simulink model "ExoskeletonControlModel"  (R2022b)
settings: Solver=ode3  StartTime=0.0  StopTime=inf  FixedStep=Ts  RelTol=1e-3
PreLoadFcn:
  | Ts_IO204 = 0.001;
  | 
  | if ~exist('Ts', 'var')
  | Ts = 0.001;
  | end
  | if ~exist('FPGA_Frequency', 'var')
  | FPGA_Frequency = 75000000;
  | end
  | 
  | ts_IO612 = 1e-3;
  | 
  | load('TargetReached.mat')
  | load('ActualPos_inc.mat')
model workspace (MAT data in the model file):
  DeltaData : timeseries (value not decoded)
  EC45_deg2incs = 2276
  EC60_deg2inc = 5461
  EC90_deg2incs = 7111
  Enc2rad_18bit = 2.3968e-05
  Enc2rad_19bit = 1.1984e-05
  Enc2rad_20bit = 5.9921e-06
  GiulioModel : robotics.RigidBodyTree (value not decoded)
  Giulio_Spheric_model : robotics.RigidBodyTree (value not decoded)
  Offset1_ticks = 571315
  Offset2_ticks = 590938.9928
  Offset3_ticks = 457912.8279
  Offset4_ticks = 482293.9763
  Offset5_ticks = 598735.9316
  Offset_M1 = 1.12645499896
  Offset_M2 = 4.02728553608
  Offset_M3 = 5.48587511336
  Offset_M4 = 2.03717511516
  Offset_M5 = 4.4996674016
  T1_Nm : object (value not decoded)
  T2_Nm : object (value not decoded)
  TBmodel : robotics.RigidBodyTree (value not decoded)
  Ts = 0.002
  Xg : object (value not decoded)
  Yg : object (value not decoded)
  Zg : object (value not decoded)
  a2 = 0.27
  change_variable = 0
  d1 = [0 0 0 0 0 0 0 0 0 0 0 0 ... (30001 elements, 30001x1)]
  d1_1 = 0.21074
  d2 = [0 0 0 0 0 0 0 0 0 0 0 0 ... (30001 elements, 30001x1)]
  d2_1 = 0.04864
  d3 = [0 0 0 0 0 0 0 0 0 0 0 0 ... (30001 elements, 30001x1)]
  d4 = [0 0 0 0 0 0 0 0 0 0 0 0 ... (30001 elements, 30001x1)]
  d5 = [0 0 0 0 0 0 0 0 0 0 0 0 ... (30001 elements, 30001x1)]
  d6 = [0 0 0 0 0 0 0 0 0 0 0 0 ... (30001 elements, 30001x1)]
  ee_x = -0.2852
  ee_y = -0.3683
  ee_z = -0.0386
  enc2rad_EC45 = 7.6699e-06
  enc2rad_EC90 = 2.3969e-05
  k1_Nm_ticks = 0.00923
  k2_Nm_ticks = 0.0257
  k3_Nm_ticks = 0.00692
  k4_Nm_ticks = 0.00729
  k5_Nm_ticks = 0.00641
  lower_lim_m1 = -330000
  lower_lim_m2 = -235302
  lower_lim_m3 = -132865
  lower_lim_m4 = -152732
  lower_lim_m5 = -138363
  lower_lim_m6 = -200325
  m1 = 2.441408578
  m2 = 3.750007
  m3 = 1.56250298
  m4 = 1.56250298
  m5 = 1.56250298
  m6 = 1.56250298
  n_oversampling = 8
  offset_sea_1 = 0.5547
  offset_sea_2 = 2.8595
  offset_sea_3 = 3.5058
  offset_sea_4 = 2.8586
  offset_sea_5 = 2.8736
  params : AKSIM (value not decoded)
  pos_th_neg = -180000
  pos_th_pos = 180000
  q1 = -1819347
  q2 = -196752
  q3 = -596465
  q4 = -556807
  q5 = -573932
  q6 = -489063
  sine = [0 0.187999937334 0.751998997352 1.69199492401 3.0079839574 4.6999608335 6.76791878442 9.21184953835 12.0317433196 15.2275888485 18.7993733417 22.7470825122 ... (12501 elements, 12501x1)]
  start : object (value not decoded)
  switch_admittance = 1
  t1 : object (value not decoded)
  t2 : object (value not decoded)
  torsionalStiffnes_M1 = 384.88
  torsionalStiffnes_M2 = 1500
  torsionalStiffnes_M3 = 901.97
  torsionalStiffnes_M4 = 950.86
  torsionalStiffnes_M5 = 930
  torsionalStiffnes_M6 = 914
  upper_lim_m1 = 340000
  upper_lim_m2 = 95467
  upper_lim_m3 = 164951
  upper_lim_m4 = 210607
  upper_lim_m5 = 252595
  upper_lim_m6 = 96694
  vel_th_neg = -100
  vel_th_pos = 100
  x = 0
undefined symbols (not defined in the file): C, DiscIntNeverNeededParam
libraries: canmsglib x285, speedgoatlib_IO614 x245, simulink x26, slrealtimeloglib x9, simulink_extras x6, robotmaniplib x6
(part 12 of 13)

== stateflow chart ExoskeletonControlModel/DataProcessing/Working_Chart ==
  state Sleep
    en:
    Working_Chart_state=1
    EnableCST=0
    EnableCSPM5=0
    EnableCSPM6=0
    EnableLR_CSP=0
    goal_m1=0
    goal_m2=0
    goal_m3=0
    goal_m4=0
    goal_m5=0
    goal_m6=0
  state Transparency
    state Block_not_recorded_joints
      state ST1_set_CSP_M1 [parallel]
        settings: executionOrder=1
      state ST1_set_CSP_M6 [parallel]
        settings: executionOrder=2
    state Learn
      state Initialize
        en:
        Working_Chart_state=12
        Spring_m6=0
        Spring_m5=0
        Spring_m4=0
        Spring_m3=0
        i=1;
        buffer5(:,1)=0;
        LearnedMovement5(:,1)=0;
        buffer4(:,1)=0;
        LearnedMovement4(:,1)=0;
        buffer3(:,1)=0;
        LearnedMovement3(:,1)=0;
      state writeRegister
        en:
        LearnedMovement5(k,1)=buffer5(k,1);
        LearnedMovement4(k,1)=buffer4(k,1);
        LearnedMovement3(k,1)=buffer3(k,1);
        mov_lenght=i;
        Working_Chart_state=11
      state Recording
        en:
        Start_m1=1
        Start_m2=1
        Start_m3=1
        Start_m4=1
        Start_m5=1
        Start_m6=1
        Working_Chart_state=4
        buffer5(i,1)=ActualPos_inc.p5;
        buffer4(i,1)=ActualPos_inc.p4;
        buffer3(i,1)=ActualPos_inc.p3;
      (default) -> Initialize
      writeRegister -> writeRegister [order 2] : [after(0.002,sec)]{k=k+1}
      Recording -> writeRegister [order 1] : [(hasChangedTo(Mode_selector,8))||(i>9998)]{k=1}
      Initialize -> Recording : [Mode_selector==7]{EnableCST=1}
      Recording -> Recording [order 2] : [after(0.002,sec)]{i=i+1}
    state TransparencyMode
      state EnablePIDs
        Start_m1=1
        Start_m2=1
        Start_m3=1
        Start_m4=1
        Start_m5=1
        Start_m6=1
      state TransparencyActive
        Working_Chart_state=4
        Spring_m6=0
        Spring_m5=0
        Spring_m4=0
        Spring_m3=0
      state WorkingInTrasparency
      (default) -> TransparencyActive
      Transparency.TransparencyMode.EnablePIDs -> WorkingInTrasparency
      TransparencyActive -> Transparency.TransparencyMode.EnablePIDs : {EnableCST=1}
    state ResetState
    state SET_MODE
      state ST1_set_CST_M1 [parallel]
        settings: executionOrder=1
      state ST1_set_CSP_M2 [parallel]
        settings: executionOrder=2
      state ST1_set_CST_M3 [parallel]
        settings: executionOrder=3
      state ST1_set_CST_M4 [parallel]
        settings: executionOrder=4
      state ST1_set_CST_M5 [parallel]
        settings: executionOrder=5
      state ST1_set_CST_M6 [parallel]
        settings: executionOrder=6
    state ImpedanceMode
      state ShoulderFlexion
        state ST1_set_CSP_M4 [parallel]
          settings: executionOrder=1
        state ST1_set_CSP_M3 [parallel]
          settings: executionOrder=2
        state ST1_set_CSP_M6 [parallel]
          settings: executionOrder=3
      state EnablePIDs
        en:
        reset_count_M5=1
        Start_m1=1
        Start_m2=1
        Start_m3=1
        Start_m4=1
        Start_m5=1
        Start_m6=1
      state WorkingInImpedance
      (default) -> ShoulderFlexion : {Working_Chart_state=5;}
      Transparency.ImpedanceMode.EnablePIDs -> WorkingInImpedance
      ShoulderFlexion -> Transparency.ImpedanceMode.EnablePIDs : {EnableCST=1}
    state L_R_CSP
      en:
      EnableLR_CSP=1;
      Working_Chart_state=13
    state GoToExerciseHome
      Working_Chart_state=6
      EnableCST=0
      EnableCSPM5=0
      EnableCSPM6=0
      EnableLR_CSP=0
      goal_m1=0
      goal_m2=0
      goal_m3=0
      goal_m4=0
      goal_m5=0
      goal_m6=0
      state GoHome_M1 [parallel]
        settings: executionOrder=1
        state ST1_set_PPM_M1
        state ST2_Switch_on_Enable_M1
        state ST3_send_target_pos_M1
        state ST4_Abs_ref_start_immediatly_M1
        state Wait_M1
        state Reached_M1
          goal_m1=1
        (default) -> Transparency.GoToExerciseHome.GoHome_M1.ST1_set_PPM_M1
        Transparency.GoToExerciseHome.GoHome_M1.ST1_set_PPM_M1 -> Transparency.GoToExerciseHome.GoHome_M1.ST2_Switch_on_Enable_M1
        Transparency.GoToExerciseHome.GoHome_M1.ST2_Switch_on_Enable_M1 -> Transparency.GoToExerciseHome.GoHome_M1.ST3_send_target_pos_M1
        Transparency.GoToExerciseHome.GoHome_M1.ST3_send_target_pos_M1 -> Transparency.GoToExerciseHome.GoHome_M1.ST4_Abs_ref_start_immediatly_M1
        Transparency.GoToExerciseHome.GoHome_M1.ST4_Abs_ref_start_immediatly_M1 -> Transparency.GoToExerciseHome.GoHome_M1.Wait_M1
        Transparency.GoToExerciseHome.GoHome_M1.Wait_M1 -> Transparency.GoToExerciseHome.GoHome_M1.Reached_M1 : [TargetReached.m1=="Target reached"]
      state GoHome_M2 [parallel]
        settings: executionOrder=2
        state ST1_set_PPM_M2
        state ST2_Switch_on_Enable_M2
        state ST3_send_target_pos_M2
        state ST4_Abs_ref_start_immediatly_M2
        state Wait_M2
        state Reached_M1
          goal_m2=1
        (default) -> Transparency.GoToExerciseHome.GoHome_M2.ST1_set_PPM_M2
        Transparency.GoToExerciseHome.GoHome_M2.ST1_set_PPM_M2 -> Transparency.GoToExerciseHome.GoHome_M2.ST2_Switch_on_Enable_M2
        Transparency.GoToExerciseHome.GoHome_M2.ST2_Switch_on_Enable_M2 -> Transparency.GoToExerciseHome.GoHome_M2.ST3_send_target_pos_M2
        Transparency.GoToExerciseHome.GoHome_M2.ST3_send_target_pos_M2 -> Transparency.GoToExerciseHome.GoHome_M2.ST4_Abs_ref_start_immediatly_M2
        Transparency.GoToExerciseHome.GoHome_M2.ST4_Abs_ref_start_immediatly_M2 -> Transparency.GoToExerciseHome.GoHome_M2.Wait_M2
        Transparency.GoToExerciseHome.GoHome_M2.Wait_M2 -> Transparency.GoToExerciseHome.GoHome_M2.Reached_M1 : [TargetReached.m2=="Target reached"]
      state GoHome_M3 [parallel]
        settings: executionOrder=3
        state ST1_set_PPM_M3
        state ST2_Switch_on_Enable_M3
        state ST3_send_target_pos_M3
        state ST4_Abs_ref_start_immediatly_M3
        state Wait_M3
        state Reached_M3
          goal_m3=1
        (default) -> Transparency.GoToExerciseHome.GoHome_M3.ST1_set_PPM_M3
        Transparency.GoToExerciseHome.GoHome_M3.ST1_set_PPM_M3 -> Transparency.GoToExerciseHome.GoHome_M3.ST2_Switch_on_Enable_M3
        Transparency.GoToExerciseHome.GoHome_M3.ST2_Switch_on_Enable_M3 -> Transparency.GoToExerciseHome.GoHome_M3.ST3_send_target_pos_M3
        Transparency.GoToExerciseHome.GoHome_M3.ST3_send_target_pos_M3 -> Transparency.GoToExerciseHome.GoHome_M3.ST4_Abs_ref_start_immediatly_M3
        Transparency.GoToExerciseHome.GoHome_M3.ST4_Abs_ref_start_immediatly_M3 -> Transparency.GoToExerciseHome.GoHome_M3.Wait_M3
        Transparency.GoToExerciseHome.GoHome_M3.Wait_M3 -> Transparency.GoToExerciseHome.GoHome_M3.Reached_M3 : [TargetReached.m3=="Target reached"]
      state GoHome_M4 [parallel]
        settings: executionOrder=4
        state ST1_set_PPM_M4
        state ST2_Switch_on_Enable_M4
        state ST3_send_target_pos_M4
        state ST4_Abs_ref_start_immediatly_M4
        state Wait_M4
        state Reached_M4
          goal_m4=1
        state ST3_send_target_pos_M4_abd
        (default) -> Transparency.GoToExerciseHome.GoHome_M4.ST1_set_PPM_M4
        Transparency.GoToExerciseHome.GoHome_M4.ST1_set_PPM_M4 -> Transparency.GoToExerciseHome.GoHome_M4.ST2_Switch_on_Enable_M4
        Transparency.GoToExerciseHome.GoHome_M4.ST2_Switch_on_Enable_M4 -> Transparency.GoToExerciseHome.GoHome_M4.ST3_send_target_pos_M4 [order 1] : [(Mode_selector==4)||(Mode_selector==5)||(Mode_selector==9)]
        Transparency.GoToExerciseHome.GoHome_M4.ST3_send_target_pos_M4 -> (junction 459)
        (junction 459) -> Transparency.GoToExerciseHome.GoHome_M4.ST4_Abs_ref_start_immediatly_M4
        Transparency.GoToExerciseHome.GoHome_M4.ST4_Abs_ref_start_immediatly_M4 -> Transparency.GoToExerciseHome.GoHome_M4.Wait_M4
        Transparency.GoToExerciseHome.GoHome_M4.Wait_M4 -> Transparency.GoToExerciseHome.GoHome_M4.Reached_M4 : [TargetReached.m4=="Target reached"]
        ST3_send_target_pos_M4_abd -> (junction 459)
        Transparency.GoToExerciseHome.GoHome_M4.ST2_Switch_on_Enable_M4 -> ST3_send_target_pos_M4_abd [order 2] : [Mode_selector==6]
      state GoHome_M5 [parallel]
        settings: executionOrder=5
        state ST1_set_PPM_M5
        state ST2_Switch_on_Enable_M5
        state ST3_send_target_pos_M5
        state ST4_Abs_ref_start_immediatly_M5
        state Wait_M5
        state Reached_M5
          goal_m5=1
        (default) -> Transparency.GoToExerciseHome.GoHome_M5.ST1_set_PPM_M5
        Transparency.GoToExerciseHome.GoHome_M5.ST1_set_PPM_M5 -> Transparency.GoToExerciseHome.GoHome_M5.ST2_Switch_on_Enable_M5
        Transparency.GoToExerciseHome.GoHome_M5.ST2_Switch_on_Enable_M5 -> Transparency.GoToExerciseHome.GoHome_M5.ST3_send_target_pos_M5
        Transparency.GoToExerciseHome.GoHome_M5.ST3_send_target_pos_M5 -> Transparency.GoToExerciseHome.GoHome_M5.ST4_Abs_ref_start_immediatly_M5
        Transparency.GoToExerciseHome.GoHome_M5.ST4_Abs_ref_start_immediatly_M5 -> Transparency.GoToExerciseHome.GoHome_M5.Wait_M5
        Transparency.GoToExerciseHome.GoHome_M5.Wait_M5 -> Transparency.GoToExerciseHome.GoHome_M5.Reached_M5 : [TargetReached.m5=="Target reached"]
      state GoHome_M6 [parallel]
        settings: executionOrder=6
        state ST1_set_PPM_M6
        state ST2_Switch_on_Enable_M6
        state ST3_send_target_pos_M6
        state ST4_Abs_ref_start_immediatly_M6
        state Wait_M6
        state Reached_M6
          goal_m6=1
        (default) -> Transparency.GoToExerciseHome.GoHome_M6.ST1_set_PPM_M6
        Transparency.GoToExerciseHome.GoHome_M6.ST1_set_PPM_M6 -> Transparency.GoToExerciseHome.GoHome_M6.ST2_Switch_on_Enable_M6
        Transparency.GoToExerciseHome.GoHome_M6.ST2_Switch_on_Enable_M6 -> Transparency.GoToExerciseHome.GoHome_M6.ST3_send_target_pos_M6
        Transparency.GoToExerciseHome.GoHome_M6.ST3_send_target_pos_M6 -> Transparency.GoToExerciseHome.GoHome_M6.ST4_Abs_ref_start_immediatly_M6
        Transparency.GoToExerciseHome.GoHome_M6.ST4_Abs_ref_start_immediatly_M6 -> Transparency.GoToExerciseHome.GoHome_M6.Wait_M6
        Transparency.GoToExerciseHome.GoHome_M6.Wait_M6 -> Transparency.GoToExerciseHome.GoHome_M6.Reached_M6 : [TargetReached.m6=="Target reached"]
    state LowAssistance
      Spring_m5=13
      Spring_m4=15
      Spring_m3=13
    state Set_CST_M5_ShoulderFlexion1
      Working_Chart_state=13
      state ST1_set_CST_M5 [parallel]
        settings: executionOrder=1
      state ST1_set_CST_M3 [parallel]
        settings: executionOrder=2
      state ST1_set_CST_M4 [parallel]
        settings: executionOrder=3
    state MediumAssistance
      Spring_m5=25
      Spring_m4=20
      Spring_m3=20
    state HighAssistance
      Spring_m5=35
      Spring_m4=30
      Spring_m3=30
    state Set_CST_M5_ShoulderFlexion
      Working_Chart_state=6
      state ST1_set_CST_M5
    state Enable
      en:
      Start_m1=1
      Start_m2=1
      Start_m3=1
      Start_m4=1
      Start_m5=1
      Start_m6=1
    state SetCSPforALL
      state ST1_set_CSP_M1 [parallel]
        settings: executionOrder=1
      state ST1_set_CSP_M2 [parallel]
        settings: executionOrder=2
      state ST1_set_CSP_M3 [parallel]
        settings: executionOrder=3
      state ST1_set_CST_M5 [parallel]
        settings: executionOrder=6
      state ST1_set_CSP_M4 [parallel]
        settings: executionOrder=4
      state ST1_set_CSP_M6 [parallel]
        settings: executionOrder=5
    state LowAssistance2
      Spring_m5=10
    state WIP_Exercise
    state MediumAssistance2
      Spring_m5=30
    state HighAssistance2
      Spring_m5=55
    state ENABLE_RIGID_CONTROL_M5
      en:
      Working_Chart_state=6
      EnableCSPM5=1
      EnableCSPM6=0
    state Set_CST_M6_ElbowFlexion
      Working_Chart_state=7
      state ST1_set_CST_M6
    state ExerciseEnded
    state ENABLE_RIGID_CONTROL_M6
      en:
      Working_Chart_state=7
      EnableCSPM5=0
      EnableCSPM6=1
    state LowAssistance1
      Spring_m6=10
    state MediumAssistance1
      Spring_m6=20
    state HighAssistance1
      Spring_m6=30
    Block_not_recorded_joints -> Learn : {i=1;}
    SET_MODE -> Block_not_recorded_joints [order 1] : [Mode_selector==7]
    (default) -> ResetState
    SET_MODE -> TransparencyMode [order 2] : [Mode_selector==2]
    ResetState -> SET_MODE [order 1] : [(Mode_selector==2)||(Mode_selector==3)||(Mode_selector==7)]
    SET_MODE -> ImpedanceMode [order 3] : [Mode_selector==3]
    ResetState -> GoToExerciseHome [order 2] : [(Mode_selector==4)||(Mode_selector==5)||(Mode_selector==6)]
    ResetState -> SetCSPforALL [order 3] : [(Mode_selector==9)]{EnableCST=0}
    WorkingInImpedance -> (junction 436) : [hasChangedFrom(SignalEnded,0)]
    SetCSPforALL -> L_R_CSP [order 6] : [(Mode_selector==9)&&(AssistanceLevel==4)]
    L_R_CSP -> (junction 541)
    LowAssistance -> (junction 506)
    Set_CST_M5_ShoulderFlexion1 -> LowAssistance [order 1] : [AssistanceLevel==1]
    MediumAssistance -> (junction 506)
    (junction 506) -> (junction 451)
    HighAssistance -> (junction 506)
    Set_CST_M5_ShoulderFlexion1 -> MediumAssistance [order 2] : [AssistanceLevel==2]
    SetCSPforALL -> Set_CST_M5_ShoulderFlexion1 [order 3] : [(Mode_selector==9)&&(AssistanceLevel<4)]
    Set_CST_M5_ShoulderFlexion1 -> HighAssistance [order 3] : [AssistanceLevel==3]
    Set_CST_M5_ShoulderFlexion -> LowAssistance2 [order 2] : [AssistanceLevel==1]
    SetCSPforALL -> Set_CST_M5_ShoulderFlexion [order 1] : [((Mode_selector==4)||(Mode_selector==6))&&AssistanceLevel<4]
    (junction 528) -> (junction 451)
    LowAssistance2 -> (junction 528)
    HighAssistance2 -> (junction 528)
    MediumAssistance2 -> (junction 528)
    (junction 451) -> Enable : {EnableCST=1}
    Enable -> (junction 541)
    (junction 541) -> WIP_Exercise
    ENABLE_RIGID_CONTROL_M6 -> (junction 541)
    (junction 527) -> (junction 451)
    ENABLE_RIGID_CONTROL_M5 -> (junction 541)
    WIP_Exercise -> ExerciseEnded : [hasChangedFrom(SignalEnded,0)]{Working_Chart_state=8}
    Set_CST_M5_ShoulderFlexion -> HighAssistance2 [order 1] : [AssistanceLevel==3]
    Set_CST_M5_ShoulderFlexion -> MediumAssistance2 [order 3] : [AssistanceLevel==2]
    GoToExerciseHome -> SetCSPforALL : [(goal_m1+goal_m2+goal_m3+goal_m4+goal_m5+goal_m6)==6]
    SetCSPforALL -> Set_CST_M6_ElbowFlexion [order 2] : [(Mode_selector==5)&&AssistanceLevel<4]
    SetCSPforALL -> ENABLE_RIGID_CONTROL_M5 [order 4] : [((Mode_selector==4)||(Mode_selector==6))&&AssistanceLevel==4]
    SetCSPforALL -> ENABLE_RIGID_CONTROL_M6 [order 5] : [(Mode_selector==5)&&AssistanceLevel==4]
    Set_CST_M6_ElbowFlexion -> LowAssistance1 [order 1] : [AssistanceLevel==1]
    Set_CST_M6_ElbowFlexion -> HighAssistance1 [order 3] : [AssistanceLevel==3]
    Set_CST_M6_ElbowFlexion -> MediumAssistance1 [order 2] : [AssistanceLevel==2]
    ExerciseEnded -> (junction 436) : after(5,sec)
    LowAssistance1 -> (junction 527)
    MediumAssistance1 -> (junction 527)
    HighAssistance1 -> (junction 527)
  state GoHome
    Working_Chart_state=2
    reset_count_M5=0
    EnableCST=0
    EnableCSPM5=0
    EnableCSPM6=0
    EnableLR_CSP=0
    goal_m1=0
    goal_m2=0
    goal_m3=0
    goal_m4=0
    goal_m5=0
    goal_m6=0
    state GoHome_M1 [parallel]
      settings: executionOrder=1
      state ST1_set_PPM_M1
      state ST2_Switch_on_Enable_M1
      state ST3_send_target_pos_M1
      state ST4_Abs_ref_start_immediatly_M1
      state Wait_M1
      state Reached_M1
        goal_m1=1
      (default) -> GoHome.GoHome_M1.ST1_set_PPM_M1
      GoHome.GoHome_M1.ST1_set_PPM_M1 -> GoHome.GoHome_M1.ST2_Switch_on_Enable_M1
      GoHome.GoHome_M1.ST2_Switch_on_Enable_M1 -> GoHome.GoHome_M1.ST3_send_target_pos_M1
      GoHome.GoHome_M1.ST3_send_target_pos_M1 -> GoHome.GoHome_M1.ST4_Abs_ref_start_immediatly_M1
      GoHome.GoHome_M1.ST4_Abs_ref_start_immediatly_M1 -> GoHome.GoHome_M1.Wait_M1
      GoHome.GoHome_M1.Wait_M1 -> GoHome.GoHome_M1.Reached_M1 : [TargetReached.m1=="Target reached"]
    state GoHome_M2 [parallel]
      settings: executionOrder=2
      state ST1_set_PPM_M2
      state ST2_Switch_on_Enable_M2
      state ST3_send_target_pos_M2
      state ST4_Abs_ref_start_immediatly_M2
      state Wait_M2
      state Reached_M1
        goal_m2=1
      (default) -> GoHome.GoHome_M2.ST1_set_PPM_M2
      GoHome.GoHome_M2.ST1_set_PPM_M2 -> GoHome.GoHome_M2.ST2_Switch_on_Enable_M2
      GoHome.GoHome_M2.ST2_Switch_on_Enable_M2 -> GoHome.GoHome_M2.ST3_send_target_pos_M2
      GoHome.GoHome_M2.ST3_send_target_pos_M2 -> GoHome.GoHome_M2.ST4_Abs_ref_start_immediatly_M2
      GoHome.GoHome_M2.ST4_Abs_ref_start_immediatly_M2 -> GoHome.GoHome_M2.Wait_M2
      GoHome.GoHome_M2.Wait_M2 -> GoHome.GoHome_M2.Reached_M1 : [TargetReached.m2=="Target reached"]
    state GoHome_M3 [parallel]
      settings: executionOrder=3
      state ST1_set_PPM_M3
      state ST2_Switch_on_Enable_M3
      state ST3_send_target_pos_M3
      state ST4_Abs_ref_start_immediatly_M3
      state Wait_M3
      state Reached_M3
        goal_m3=1
      (default) -> GoHome.GoHome_M3.ST1_set_PPM_M3
      GoHome.GoHome_M3.ST1_set_PPM_M3 -> GoHome.GoHome_M3.ST2_Switch_on_Enable_M3
      GoHome.GoHome_M3.ST2_Switch_on_Enable_M3 -> GoHome.GoHome_M3.ST3_send_target_pos_M3
      GoHome.GoHome_M3.ST3_send_target_pos_M3 -> GoHome.GoHome_M3.ST4_Abs_ref_start_immediatly_M3
      GoHome.GoHome_M3.ST4_Abs_ref_start_immediatly_M3 -> GoHome.GoHome_M3.Wait_M3
      GoHome.GoHome_M3.Wait_M3 -> GoHome.GoHome_M3.Reached_M3 : [TargetReached.m3=="Target reached"]
    state GoHome_M4 [parallel]
      settings: executionOrder=4
      state ST1_set_PPM_M4
      state ST2_Switch_on_Enable_M4
      state ST3_send_target_pos_M4
      state ST4_Abs_ref_start_immediatly_M4
      state Wait_M4
      state Reached_M4
        goal_m4=1
      (default) -> GoHome.GoHome_M4.ST1_set_PPM_M4
      GoHome.GoHome_M4.ST1_set_PPM_M4 -> GoHome.GoHome_M4.ST2_Switch_on_Enable_M4
      GoHome.GoHome_M4.ST2_Switch_on_Enable_M4 -> GoHome.GoHome_M4.ST3_send_target_pos_M4
      GoHome.GoHome_M4.ST3_send_target_pos_M4 -> GoHome.GoHome_M4.ST4_Abs_ref_start_immediatly_M4
      GoHome.GoHome_M4.ST4_Abs_ref_start_immediatly_M4 -> GoHome.GoHome_M4.Wait_M4
      GoHome.GoHome_M4.Wait_M4 -> GoHome.GoHome_M4.Reached_M4 : [TargetReached.m4=="Target reached"]
    state GoHome_M5 [parallel]
      settings: executionOrder=5
      state ST1_set_PPM_M5
      state ST2_Switch_on_Enable_M5
      state ST3_send_target_pos_M5
      state ST4_Abs_ref_start_immediatly_M5
      state Wait_M5
      state Reached_M5
        goal_m5=1
      (default) -> GoHome.GoHome_M5.ST1_set_PPM_M5
      GoHome.GoHome_M5.ST1_set_PPM_M5 -> GoHome.GoHome_M5.ST2_Switch_on_Enable_M5
      GoHome.GoHome_M5.ST2_Switch_on_Enable_M5 -> GoHome.GoHome_M5.ST3_send_target_pos_M5
      GoHome.GoHome_M5.ST3_send_target_pos_M5 -> GoHome.GoHome_M5.ST4_Abs_ref_start_immediatly_M5
      GoHome.GoHome_M5.ST4_Abs_ref_start_immediatly_M5 -> GoHome.GoHome_M5.Wait_M5
      GoHome.GoHome_M5.Wait_M5 -> GoHome.GoHome_M5.Reached_M5 : [TargetReached.m5=="Target reached"]
    state GoHome_M6 [parallel]
      settings: executionOrder=6
      state ST1_set_PPM_M6
      state ST2_Switch_on_Enable_M6
      state ST3_send_target_pos_M6
      state ST4_Abs_ref_start_immediatly_M6
      state Wait_M6
      state Reached_M6
        goal_m6=1
      (default) -> GoHome.GoHome_M6.ST1_set_PPM_M6
      GoHome.GoHome_M6.ST1_set_PPM_M6 -> GoHome.GoHome_M6.ST2_Switch_on_Enable_M6
      GoHome.GoHome_M6.ST2_Switch_on_Enable_M6 -> GoHome.GoHome_M6.ST3_send_target_pos_M6
      GoHome.GoHome_M6.ST3_send_target_pos_M6 -> GoHome.GoHome_M6.ST4_Abs_ref_start_immediatly_M6
      GoHome.GoHome_M6.ST4_Abs_ref_start_immediatly_M6 -> GoHome.GoHome_M6.Wait_M6
      GoHome.GoHome_M6.Wait_M6 -> GoHome.GoHome_M6.Reached_M6 : [TargetReached.m6=="Target reached"]
  state HomePositionActive
    Working_Chart_state=3
  state FaultManagment
    Working_Chart_state=10
    EnableCST=0
    EnableCSPM5=0
    EnableCSPM6=0
    goal_m1=0
    goal_m2=0
    goal_m3=0
    goal_m4=0
    goal_m5=0
    goal_m6=0
    Start_m1=0
    Start_m2=0
    Start_m3=0
    Start_m4=0
    Start_m5=0
    Start_m6=0
  writeRegister -> GoHome [order 1] : [k>=i]
  (default) -> Sleep
  (junction 189) -> Sleep
  Sleep -> GoHome : [hasChangedTo(Homing_all_motors,1)]
  Transparency -> (junction 189) [order 1] : [hasChangedTo(Homing_all_motors,0)]
  GoHome -> (junction 189) [order 2] : [hasChangedTo(Homing_all_motors,0)]
  HomePositionActive -> (junction 189) [order 2] : [hasChangedTo(Homing_all_motors,0)]
  HomePositionActive -> Transparency [order 1] : [(hasChangedTo(Mode_selector,2))||(hasChangedTo(Mode_selector,3))||(hasChangedTo(Mode_selector,4))||(hasChangedTo(Mode_selector,5))||(hasChangedTo(Mode_selector,6))||(hasChangedTo(Mode_selector,9))||(hasChangedTo(Mode_selector,7))]
  GoHome -> HomePositionActive [order 1] : [(goal_m1+goal_m2+goal_m3+goal_m4+goal_m5+goal_m6)==6]
  HomePositionActive -> (junction 285) [order 3]
  Transparency -> GoHome [order 3] : [hasChangedTo(Mode_selector,1)]
  Transparency -> (junction 285) [order 2]
  (junction 285) -> FaultManagment : [Fault_error==1]
  GoHome -> (junction 285) [order 3]
  (junction 436) -> GoHome
  FaultManagment -> GoHome : [hasChangedTo(Mode_selector,100) && Fault_error==0]
  data: sf_internal_action_state_placeholder_data local double size=1 =0; sf_internal_action_state_placeholder_data local double size=1 =0; sf_internal_action_state_placeholder_data local double size=1 =0; sf_internal_action_state_placeholder_data local double size=1 =0; sf_internal_action_state_placeholder_data local double size=1 =0; sf_internal_action_state_placeholder_data local double size=1 =0; sf_internal_action_state_placeholder_data local double size=1 =0; sf_internal_action_state_placeholder_data local double size=1 =0; sf_internal_action_state_placeholder_data local double size=1 =0; sf_internal_action_state_placeholder_data local double size=1 =0; sf_internal_action_state_placeholder_data local double size=1 =0; sf_internal_action_state_placeholder_data local double size=1 =0; sf_internal_action_state_placeholder_data local double size=1 =0; sf_internal_action_state_placeholder_data local double size=1 =0; sf_internal_action_state_placeholder_data local double size=1 =0; sf_internal_action_state_placeholder_data local double size=1 =0; sf_internal_action_state_placeholder_data local double size=1 =0; sf_internal_action_state_placeholder_data local double size=1 =0; sf_internal_action_state_placeholder_data local double size=1 =0; sf_internal_action_state_placeholder_data local double size=1 =0; sf_internal_action_state_placeholder_data local double size=1 =0; sf_internal_action_state_placeholder_data local double size=1 =0; sf_internal_action_state_placeholder_data local double size=1 =0; sf_internal_action_state_placeholder_data local double size=1 =0; sf_internal_action_state_placeholder_data local double size=1 =0; sf_internal_action_state_placeholder_data local double size=1 =0; sf_internal_action_state_placeholder_data local double size=1 =0; sf_internal_action_state_placeholder_data local double size=1 =0; sf_internal_action_state_placeholder_data local double size=1 =0; sf_internal_action_state_placeholder_data local double size=1 =0; sf_internal_action_state_placeholder_data local double size=1 =0; sf_internal_action_state_placeholder_data local double size=1 =0; sf_internal_action_state_placeholder_data local double size=1 =0; sf_internal_action_state_placeholder_data local double size=1 =0; sf_internal_action_state_placeholder_data local double size=1 =0; sf_internal_action_state_placeholder_data local double size=1 =0; sf_internal_action_state_placeholder_data local double size=1 =0; sf_internal_action_state_placeholder_data local double size=1 =0; sf_internal_action_state_placeholder_data local double size=1 =0; sf_internal_action_state_placeholder_data local double size=1 =0; sf_internal_action_state_placeholder_data local double size=1 =0; sf_internal_action_state_placeholder_data local double size=1 =0; sf_internal_action_state_placeholder_data local double size=1 =0; sf_internal_action_state_placeholder_data local double size=1 =0; sf_internal_action_state_placeholder_data local double size=1 =0; sf_internal_action_state_placeholder_data local double size=1 =0; sf_internal_action_state_placeholder_data local double size=1 =0; sf_internal_action_state_placeholder_data local double size=1 =0; sf_internal_action_state_placeholder_data local double size=1 =0; sf_internal_action_state_placeholder_data local double size=1 =0; sf_internal_action_state_placeholder_data local double size=1 =0; sf_internal_action_state_placeholder_data local double size=1 =0; sf_internal_action_state_placeholder_data local double size=1 =0; sf_internal_action_state_placeholder_data local double size=1 =0; sf_internal_action_state_placeholder_data local double size=1 =0; sf_internal_action_state_placeholder_data local double size=1 =0; sf_internal_action_state_placeholder_data local double size=1 =0; sf_internal_action_state_placeholder_data local double size=1 =0; sf_internal_action_state_placeholder_data local double size=1 =0; sf_internal_action_state_placeholder_data local double size=1 =0; sf_internal_action_state_placeholder_data local double size=1 =0; sf_internal_action_state_placeholder_data local double size=1 =0; sf_internal_action_state_placeholder_data local double size=1 =0; sf_internal_action_state_placeholder_data local double size=1 =0; sf_internal_action_state_placeholder_data local double size=1 =0; sf_internal_action_state_placeholder_data local double size=1 =0; sf_internal_action_state_placeholder_data local double size=1 =0; sf_internal_action_state_placeholder_data local double size=1 =0; sf_internal_action_state_placeholder_data local double size=1 =0; sf_internal_action_state_placeholder_data local double size=1 =0; sf_internal_action_state_placeholder_data local double size=1 =0; sf_internal_action_state_placeholder_data local double size=1 =0; Mode_selector input; AssistanceLevel input; Homing_all_motors input; EnableCST output; TargetReached input Bus: TargetReached; goal_m1 local; goal_m2 local; goal_m3 local; goal_m4 local; goal_m5 local; goal_m6 local; Working_Chart_state output; Start_m1 data_store_memory; Start_m2 data_store_memory; Start_m3 data_store_memory; Start_m4 data_store_memory; Start_m5 data_store_memory; Start_m6 data_store_memory; reset_count_M5 data_store_memory; Fault_error input; ActualPos_inc input; SignalEnded input; buffer5 data_store_memory; i local; LearnedMovement5 data_store_memory; mov_lenght output; k local; Spring_m5 data_store_memory; Spring_m6 data_store_memory; LearnedMovement3 data_store_memory; buffer3 data_store_memory; LearnedMovement4 data_store_memory; buffer4 data_store_memory; Spring_m3 data_store_memory; Spring_m4 data_store_memory; EnableCSPM5 output; EnableCSPM6 output; EnableLR_CSP output

== matlab function ExoskeletonControlModel/DataProcessing/Subsystem/MATLAB Function ==
  data: u input; y output
function y = fcn(u)

y = u(1:3,4);

== matlab function ExoskeletonControlModel/DataProcessing/Subsystem/MATLAB Function1 ==
  data: u input; y output; x input
function y = fcn(u,x)

y = u*x;

== matlab function ExoskeletonControlModel/DataProcessing/Subsystem/MATLAB Function2 ==
  data: u input; y output
function y = fcn(u)
rot05=[0.0512 -0.8936 0.4460; 
-0.0944 0.4403 0.8929; 
-0.9942 -0.0878 -0.0618];

rot2=[0.0512 -0.0944 -0.9942;
-0.8936 0.4403 -0.0878;
0.4460 0.8929 -0.0618];


rot = u(1:3,1:3);
y=rotm2eul(rot,"ZYX")

== matlab function ExoskeletonControlModel/DataProcessing/CST_trasparency/CST_control/MOTOR4/Subsystem1/MATLAB Function2 ==
  data: sz input; signal input; count input; cnt output; reset input; signal_ended output
function [cnt, signal_ended] = fcn(sz, signal,count, reset)
signal_size = size(signal);
signal_size=signal_size(1);

if (count<sz && reset==0)
    cnt=count;
    signal_ended=0;
elseif (count>sz && reset==0)
    cnt=sz;
    signal_ended=1;
elseif reset==1
    cnt=1;
    signal_ended=0;
else
    cnt=count;
    signal_ended=0;
end

== stateflow chart ExoskeletonControlModel/DataProcessing/CST_trasparency/CST_control/MOTOR3/impedance_values_safe_zones ==
  state SafeZone_low
    state active
      y=1
      dx1=(theta-theta_low)/2276;
      new_target_torque=-k1*dx1-beta*speed
    state hard
      y=2
      dx2=(theta-theta_low_hard)/2276
      dx1=(theta-theta_low)/2276
      new_target_torque=-k1*dx1-5*k2*dx2-beta*speed;
    (default) -> SafeZone_low.active
    SafeZone_low.active -> SafeZone_low.hard : [theta < theta_low_hard]
    SafeZone_low.hard -> SafeZone_low.active : [theta >= theta_low_hard]
  state SafeZone_high
    state active
      y=5
      dx1=(theta-theta_high)/2276
      new_target_torque=-k1*dx1-beta*speed
    state hard
      y=6
      dx2=(theta-theta_high_hard)/2276
      dx1=(theta-theta_high)/2276
      new_target_torque=-k1*dx1-5*k2*dx2-beta*speed;
    (default) -> SafeZone_high.active
    SafeZone_high.active -> SafeZone_high.hard : [theta > theta_high_hard]
    SafeZone_high.hard -> SafeZone_high.active : [theta <= theta_high_hard]
  state Transparency
    en:
    k1=0.1
    k2=2
    beta=0.05
    ZH_tau_max=1
    ZL_tau_max=1
    du:
    y = 0
    new_target_torque=0
  (default) -> Transparency
  Transparency -> SafeZone_low [order 1] : [theta < theta_low]
  Transparency -> SafeZone_high [order 2] : [theta > theta_high]
  SafeZone_high -> Transparency : [theta <= theta_high && (torque< ZH_tau_max) ]
  SafeZone_low -> Transparency : [theta >= theta_low && (torque< ZL_tau_max)]
  data: theta_low_hard constant double =-137417+2276*6; theta_low constant double =-137417+2276*9; torque input; theta_high_hard constant double =169503-2276*6; theta_high constant double =169503-2276*9; theta input; speed input; new_target_torque output; dx1 local; dx2 local; y output; beta local; ZH_tau_max local; ZL_tau_max local; k1 local; k2 local

== matlab function ExoskeletonControlModel/DataProcessing/Homing_State_Machine/MATLAB Function ==
  data: stat1 input; fault_error output; stat2 input; stat3 input; stat4 input; stat5 input; stat6 input
function fault_error = fcn(stat1, stat2, stat3, stat4, stat5, stat6)
if (stat1=="Fault reaction active" || stat1=="Fault"||stat1=="Fault reaction active" || stat1=="Fault"||stat2=="Fault reaction active" || stat2=="Fault"||stat3=="Fault reaction active" || stat3=="Fault"||stat4=="Fault reaction active" || stat4=="Fault"||stat5=="Fault reaction active" || stat5=="Fault"||stat6=="Fault reaction active" || stat6=="Fault")
    fault_error=1;
else
    fault_error=0;
end

== stateflow chart ExoskeletonControlModel/DataProcessing/CST_trasparency/CST_control/MOTOR3/Chart ==
  state Trasparency
    state evaluateSpeed
    state WinFriction
      beta=-0.06
    state NotSoFast
      beta=-0.013*(3000/speed)
    state MovingFree
      beta=-0.039
    NotSoFast -> WinFriction [order 2] : [speed<=300]
    (default) -> evaluateSpeed
    WinFriction -> (junction 16) [order 2]
    evaluateSpeed -> WinFriction : [speed<300]
    MovingFree -> WinFriction [order 1] : [speed<=300]
    WinFriction -> MovingFree [order 1] : [speed>=300 && speed<=1000]
    (junction 16) -> NotSoFast : [speed>1000]
    MovingFree -> (junction 16) [order 2]
    NotSoFast -> MovingFree [order 1] : [speed<=1000]
  state EvaluateState
  state AvoidEffect
    beta=0.01
  (default) -> EvaluateState
  EvaluateState -> Trasparency [order 1] : [state==4]
  EvaluateState -> AvoidEffect [order 2] : [state~=4]
  AvoidEffect -> Trasparency : [state==4]
  Trasparency -> AvoidEffect : [state~=4]
  data: state input; speed input; beta output

== stateflow chart ExoskeletonControlModel/DataProcessing/CST_trasparency/CST_control/MOTOR6/Chart ==
  state Trasparency
    state evaluateSpeed
    state WinFriction
      beta=-0.056
    state NotSoFast
      beta=-0.0215*(2000/speed)
    state MovingFree
      beta=-0.054
      %-0.028
    NotSoFast -> WinFriction [order 2] : [speed<=300]
    (default) -> evaluateSpeed
    WinFriction -> (junction 16) [order 2]
    evaluateSpeed -> WinFriction : [speed<300]
    MovingFree -> WinFriction [order 1] : [speed<=300]
    WinFriction -> MovingFree [order 1] : [speed>=300 && speed<=800]
    (junction 16) -> NotSoFast : [speed>800]
    MovingFree -> (junction 16) [order 2]
    NotSoFast -> MovingFree [order 1] : [speed<=800]
  state EvaluateState
  state AvoidEffect
    beta=0.01
  (default) -> EvaluateState
  EvaluateState -> Trasparency [order 1] : [state==4]
  EvaluateState -> AvoidEffect [order 2] : [state~=4]
  AvoidEffect -> Trasparency : [state==4]
  Trasparency -> AvoidEffect : [state~=4]
  data: state input; speed input; beta output

== stateflow chart ExoskeletonControlModel/DataProcessing/CST_trasparency/CST_control/MOTOR4/impedance_values_safe_zones ==
  state SafeZone_low
    state active
      y=1
      dx1=(theta-theta_low)/2276;
      new_target_torque=-k1*dx1-beta*speed
    state hard
      y=2
      dx2=(theta-theta_low_hard)/2276
      dx1=(theta-theta_low)/2276
      new_target_torque=-k1*dx1-5*k2*dx2-beta*speed;
    (default) -> SafeZone_low.active
    SafeZone_low.active -> SafeZone_low.hard : [theta < theta_low_hard]
    SafeZone_low.hard -> SafeZone_low.active : [theta >= theta_low_hard]
  state SafeZone_high
    state active
      y=5
      dx1=(theta-theta_high)/2276
      new_target_torque=-k1*dx1-beta*speed
    state hard
      y=6
      dx2=(theta-theta_high_hard)/2276
      dx1=(theta-theta_high)/2276
      new_target_torque=-k1*dx1-5*k2*dx2-beta*speed;
    (default) -> SafeZone_high.active
    SafeZone_high.active -> SafeZone_high.hard : [theta > theta_high_hard]
    SafeZone_high.hard -> SafeZone_high.active : [theta <= theta_high_hard]
  state Transparency
    en:
    k1=0.1
    k2=2
    beta=0.05
    ZH_tau_max=1
    ZL_tau_max=1
    du:
    y = 0
    new_target_torque=0
  (default) -> Transparency
  Transparency -> SafeZone_low [order 1] : [theta < theta_low]
  Transparency -> SafeZone_high [order 2] : [theta > theta_high]
  SafeZone_high -> Transparency : [theta <= theta_high && (torque< ZH_tau_max) ]
  SafeZone_low -> Transparency : [theta >= theta_low && (torque< ZL_tau_max)]
  data: theta_low_hard constant double =-157284+2276*6; theta_low constant double =-157284+2276*9; torque input; theta_high_hard constant double =215159-2276*6; theta_high constant double =215159-2276*9; theta input; speed input; new_target_torque output; dx1 local; dx2 local; y output; beta local; ZH_tau_max local; ZL_tau_max local; k1 local; k2 local

== stateflow chart ExoskeletonControlModel/DataProcessing/CST_trasparency/CST_control/MOTOR4/Chart ==
  state Trasparency
    state evaluateSpeed
    state WinFriction
      beta=-0.056
    state NotSoFast
      beta=-0.020*(2000/speed)
    state MovingFree
      beta=-0.050
      %0.065
    NotSoFast -> WinFriction [order 2] : [speed<=300]
    (default) -> evaluateSpeed
    WinFriction -> (junction 16) [order 2]
    evaluateSpeed -> WinFriction : [speed<300]
    MovingFree -> WinFriction [order 1] : [speed<=300]
    WinFriction -> MovingFree [order 1] : [speed>=300 && speed<=800]
    (junction 16) -> NotSoFast : [speed>800]
    MovingFree -> (junction 16) [order 2]
    NotSoFast -> MovingFree [order 1] : [speed<=800]
  state EvaluateState
  state AvoidEffect
    beta=0.01
  (default) -> EvaluateState
  EvaluateState -> Trasparency [order 1] : [state==4]
  EvaluateState -> AvoidEffect [order 2] : [state~=4]
  AvoidEffect -> Trasparency : [state==4]
  Trasparency -> AvoidEffect : [state~=4]
  data: state input; speed input; beta output

== stateflow chart ExoskeletonControlModel/DataProcessing/CST_trasparency/CST_control/MOTOR5/Chart ==
  state Trasparency
    state evaluateSpeed
    state WinFriction
      beta=-0.05
    state NotSoFast
      beta=-0.016*(3000/speed)
    state MovingFree
      beta=-0.049
    NotSoFast -> WinFriction [order 2] : [speed<=300]
    (default) -> evaluateSpeed
    WinFriction -> (junction 16) [order 2]
    evaluateSpeed -> WinFriction : [speed<300]
    MovingFree -> WinFriction [order 1] : [speed<=300]
    WinFriction -> MovingFree [order 1] : [speed>=300 && speed<=1000]
    (junction 16) -> NotSoFast : [speed>1000]
    MovingFree -> (junction 16) [order 2]
    NotSoFast -> MovingFree [order 1] : [speed<=1000]
  state EvaluateState
  state AvoidEffect
    beta=betaTest
  (default) -> EvaluateState
  EvaluateState -> Trasparency [order 1] : [state==4]
  EvaluateState -> AvoidEffect [order 2] : [state~=4]
  AvoidEffect -> Trasparency : [state==4]
  Trasparency -> AvoidEffect : [state~=4]
  data: state input; speed input; beta output; betaTest input

== stateflow chart ExoskeletonControlModel/DataProcessing/CST_trasparency/CST_control/MOTOR5/Chart1 ==
  state Compute_target
    My_target=Max*(2276);
    repeat=Repetition;
    actualTime=clock;
    Timing=Duration;
    SignalEnded=0;
  state ForwardMovement
    gotoPos=((My_target)/Timing)*(clock-actualTime)+Neutral_pos
    updown=2;
  state BackwardMovement_Target
    gotoPos=(-(My_target)/Timing)*(clock-Timing-actualTime)+(My_target+Neutral_pos)
    updown=1;
  state TrajectoryEnded
    gotoPos=Neutral_pos
    updown=0;
  state Ended
    SignalEnded=1;
    updown=0;
  (default) -> Compute_target
  Ended -> Compute_target
  Compute_target -> ForwardMovement : [hasChangedFrom(start,0)]
  ForwardMovement -> BackwardMovement_Target : [(gotoPos>(My_target+Neutral_pos)) ]
  TrajectoryEnded -> ForwardMovement [order 1] : [repeat>0 && after(2,sec)]{actualTime=clock;}
  BackwardMovement_Target -> TrajectoryEnded : [gotoPos<Neutral_pos]{repeat=repeat-1}
  TrajectoryEnded -> Ended [order 2] : [repeat==0]
  data: Max input; Neutral_pos input; clock input; gotoPos output; My_target local; start input; actualTime local; Repetition input; repeat local; Timing local; Duration input; SignalEnded output; updown output

== stateflow chart ExoskeletonControlModel/DataProcessing/CST_trasparency/CST_control/MOTOR6/Chart1 ==
  state Compute_target
    My_target=Max*(2276);
    repeat=Repetition;
    actualTime=clock;
    Timing=Duration;
    SignalEnded=0;
  state ForwardMovement
    gotoPos=((My_target)/Timing)*(clock-actualTime)+Neutral_pos
    updown_el=2;
  state BackwardMovement_Target
    gotoPos=(-(My_target)/Timing)*(clock-Timing-actualTime)+(My_target+Neutral_pos)
    updown_el=1;
  state TrajectoryEnded
    gotoPos=Neutral_pos
    updown_el=0;
  state Ended
    SignalEnded=1;
    updown_el=0;
  (default) -> Compute_target
  Ended -> Compute_target
  Compute_target -> ForwardMovement : [hasChangedFrom(start,0)]
  TrajectoryEnded -> ForwardMovement [order 1] : [repeat>0 && after(2,sec)]{actualTime=clock;}
  BackwardMovement_Target -> TrajectoryEnded : [gotoPos<Neutral_pos]{repeat=repeat-1}
  TrajectoryEnded -> Ended [order 2] : [repeat==0]
  ForwardMovement -> BackwardMovement_Target : [(gotoPos>(My_target+Neutral_pos))]
  data: Max input; Neutral_pos input; clock input; gotoPos output; My_target local; start input; actualTime local; Repetition input; repeat local; Timing local; Duration input; SignalEnded output; updown_el output

== stateflow chart ExoskeletonControlModel/DataProcessing/CST_trasparency/CST_control/MOTOR6/impedance_values_safe_zones1 ==
  state SafeZone_low
    state active
      y=1
      dx1=(theta-theta_low)/2276;
      new_target_torque=-k1*dx1-beta*speed
    state hard
      y=2
      dx2=(theta-theta_low_hard)/2276
      dx1=(theta-theta_low)/2276
      new_target_torque=-k1*dx1-5*k2*dx2-beta*speed;
    (default) -> SafeZone_low.active
    SafeZone_low.active -> SafeZone_low.hard : [theta < theta_low_hard]
    SafeZone_low.hard -> SafeZone_low.active : [theta >= theta_low_hard]
  state SafeZone_high
    state active
      y=5
      dx1=(theta-theta_high)/2276
      new_target_torque=-k1*dx1-beta*speed
    state hard
      y=6
      dx2=(theta-theta_high_hard)/2276
      dx1=(theta-theta_high)/2276
      new_target_torque=-k1*dx1-5*k2*dx2-beta*speed;
    (default) -> SafeZone_high.active
    SafeZone_high.active -> SafeZone_high.hard : [theta > theta_high_hard]
    SafeZone_high.hard -> SafeZone_high.active : [theta <= theta_high_hard]
  state Transparency
    en:
    k1=2
    k2=4
    beta=0.05
    ZH_tau_max=1
    ZL_tau_max=1
    du:
    y = 0
    new_target_torque=0
  (default) -> Transparency
  Transparency -> SafeZone_low [order 1] : [theta < theta_low]
  Transparency -> SafeZone_high [order 2] : [theta > theta_high]
  SafeZone_high -> Transparency : [theta <= theta_high && (torque< ZH_tau_max) ]
  SafeZone_low -> Transparency : [theta >= theta_low && (torque< ZL_tau_max)]
  data: theta_low_hard constant double =-204877+2276*6; theta_low constant double =-204877+2276*9; torque input; theta_high_hard constant double =101246-2276*6; theta_high constant double =101246-2276*9; theta input; speed input; new_target_torque output; dx1 local; dx2 local; y output; beta local; ZH_tau_max local; ZL_tau_max local; k1 local; k2 local

== matlab function ExoskeletonControlModel/DataProcessing/Subsystem1/MATLAB Function ==
  data: WorkingState input; selectedEndedSignal output; EndedSH input; EndedEL input; EndedLR input
function selectedEndedSignal = fcn(WorkingState,EndedSH,EndedEL, EndedLR)
if WorkingState==6
    selectedEndedSignal=EndedSH;
elseif WorkingState==13
    selectedEndedSignal=EndedLR;
elseif WorkingState==7
    selectedEndedSignal=EndedEL;
else
    selectedEndedSignal=0;
end

== matlab function ExoskeletonControlModel/DataProcessing/CST_trasparency/CST_control/MOTOR5/Subsystem1/MATLAB Function2 ==
  data: sz input; signal input; count input; cnt output; reset input; signal_ended output
function [cnt, signal_ended] = fcn(sz, signal,count, reset)
signal_size = size(signal);
signal_size=signal_size(1);

if (count<sz && reset==0)
    cnt=count;
    signal_ended=0;
elseif (count>sz && reset==0)
    cnt=sz;
    signal_ended=1;
elseif reset==1
    cnt=1;
    signal_ended=0;
else
    cnt=count;
    signal_ended=0;
end

== matlab function ExoskeletonControlModel/DataProcessing/CST_trasparency/CST_control/MOTOR5/MATLAB Function ==
  data: mode input; refPos output; RefPosShFlex input; RefPosLR input
function refPos  = fcn(mode,RefPosShFlex,RefPosLR)
if mode==4
    
    refPos=RefPosShFlex;
    
elseif mode==6
 
    refPos=RefPosShFlex;

elseif mode==9
  
    refPos=RefPosLR;
    

else
    
    refPos=0;
    
end

== matlab function ExoskeletonControlModel/DataProcessing/CST_trasparency/CST_control/MOTOR3/Subsystem1/MATLAB Function2 ==
  data: sz input; signal input; count input; cnt output; reset input; signal_ended output
function [cnt, signal_ended] = fcn(sz, signal,count, reset)
signal_size = size(signal);
signal_size=signal_size(1);

if (count<sz && reset==0)
    cnt=count;
    signal_ended=0;
elseif (count>sz && reset==0)
    cnt=sz;
    signal_ended=1;
elseif reset==1
    cnt=1;
    signal_ended=0;
else
    cnt=count;
    signal_ended=0;
end

== matlab function ExoskeletonControlModel/DataProcessing/MATLAB Function1 ==
  data: ms input; en input; y output
function y = fcn(ms, en)
if ms==4
    y=0;
else
    y=en;
end

== matlab function ExoskeletonControlModel/DataProcessing/MATLAB Function ==
  data: enCST input; y output; enCSPM5 input; enCSPm6 input; EnableLR_CSP input
function y = fcn(enCST,enCSPM5,enCSPm6, EnableLR_CSP)
if (enCST==1||enCSPM5==1||enCSPm6==1||EnableLR_CSP==1)
    y=1;
else 
    y=0;
end

== matlab function ExoskeletonControlModel/DataProcessing/Subsystem/MATLAB Function3 ==
  data: r output; p output; u input; y output
function [r,p,y] = fcn(u)

rpy=rad2deg(rotm2eul(u(1:3,1:3),"ZYX")); 
r=rpy(3);
p=rpy(2);
y=rpy(1);

== matlab function ExoskeletonControlModel/DataProcessing/Subsystem/MATLAB Function4 ==
  data: u input; y output; x input
function y = fcn(u,x)

y = u*x;
